simulink model "TV_2021"  (R2017b)
settings: Solver=VariableStepAuto  StartTime=0.0  StopTime=10.0  RelTol=1e-3
undefined symbols (not defined in the file): sigbuilder_block
libraries: simulink x6
(part 7 of 13)

== system TV_2021/Vehicle Dynamics Control 1/VDC 2018 without Longitudinal/Driver // CarBehaviours/Accelerating ==
  Throttle : Inport
  Tq_RR : Inport  Port=2
  "Tq_RL " : Inport  Port=3
  Action Port : ActionPort
  Product : Product
  Product1 : Product
  "Tq_RR " : Outport
  Tq_RL : Outport  Port=2
  Out_Throttle : Outport  Port=3
  wires:
  "Tq_RL "/1 -> Product/2
  Tq_RR/1 -> Product1/2
  Throttle/1 -> Product1/1, Product/1, Out_Throttle/1
  Product/1 -> Tq_RL/1
  Product1/1 -> "Tq_RR "/1

== system TV_2021/Vehicle Dynamics Control 1/VDC 2018 without Longitudinal/Driver // CarBehaviours/Inertia Braking ==
  Action Port : ActionPort
  Constant : Constant  Value=0
  Constant1 : Constant  Value=0
  "Tq_RR " : Outport
  Tq_RL : Outport  Port=2
  wires:
  Constant/1 -> "Tq_RR "/1
  Constant1/1 -> Tq_RL/1

== system TV_2021/Vehicle Dynamics Control 1/VDC 2018 without Longitudinal/Driver // CarBehaviours/Mech_Braking ==
  Action Port : ActionPort
  Constant : Constant  Value=0
  Constant1 : Constant  Value=0
  "Tq_RR " : Outport
  Tq_RL : Outport  Port=2
  wires:
  Constant/1 -> "Tq_RR "/1
  Constant1/1 -> Tq_RL/1

== system TV_2021/Vehicle Dynamics Control 1/VDC 2018 without Longitudinal/Driver // CarBehaviours/Regenerative+Mech Braking ==
  RegTq_RR : Inport
  RegTq_RL : Inport  Port=2
  Action Port : ActionPort
  "Tq_RR " : Outport
  Tq_RL : Outport  Port=2
  wires:
  RegTq_RL/1 -> Tq_RL/1
  RegTq_RR/1 -> "Tq_RR "/1

== system TV_2021/Vehicle Dynamics Control 1/VDC 2018 without Longitudinal/Optimization SKF & CKF/Subsystem  ==
  Derivative : Inport
  "CKF_Initial " : Inport  Port=2
  "CKF_prev " : Inport  Port=3
  Cte_CKF : Inport  Port=4
  CKF : Subsystem
  CKF_act : Outport
  wires:
  Cte_CKF/1 -> CKF/4(Cte_CKF)
  "CKF_Initial "/1 -> CKF/2(CKF_Initial)
  Derivative/1 -> CKF/1(Derivative)
  "CKF_prev "/1 -> CKF/3("CKF_prev ")
  CKF/1("CKF_act ") -> CKF_act/1

== system TV_2021/Vehicle Dynamics Control 1/VDC 2018 without Longitudinal/Wheel_to_engine/Fx_to_engineTqRL ==
  Fx : Inport
  Re : Inport  Port=2
  RT : Inport  Port=3
  Divide : Product  Inputs=*/
  Product : Product
  Tq : Outport
  wires:
  Re/1 -> Product/2
  Fx/1 -> Product/1
  RT/1 -> Divide/2
  Product/1 -> Divide/1
  Divide/1 -> Tq/1

== system TV_2021/Vehicle Dynamics Control 1/VDC 2018 without Longitudinal/Wheel_to_engine/Fx_to_engineTqRR ==
  Fx : Inport
  Re : Inport  Port=2
  RT : Inport  Port=3
  Divide : Product  Inputs=*/
  Product : Product
  Tq : Outport
  wires:
  Re/1 -> Product/2
  Fx/1 -> Product/1
  RT/1 -> Divide/2
  Product/1 -> Divide/1
  Divide/1 -> Tq/1

== system TV_2021/Vehicle Dynamics Control 2018/Steering TV 2017 with TC/Constraints/Control de Potencia  ==
  Tq_RR : Inport
  Tq_RL : Inport  Port=2
  ReductionCte : Inport  Port=3
  Action Port : ActionPort
  Add : Sum  Inputs=+-
  Add1 : Sum  Inputs=+-
  Product : Product
  Product1 : Product
  Tq_RR_out : Outport
  Tq_RL_out : Outport  Port=2
  wires:
  Tq_RR/1 -> Product/1, Add/1
  Tq_RL/1 -> Product1/1, Add1/1
  ReductionCte/1 -> Product/2, Product1/2
  Product1/1 -> Add1/2
  Product/1 -> Add/2
  Add1/1 -> Tq_RL_out/1
  Add/1 -> Tq_RR_out/1

== system TV_2021/Vehicle Dynamics Control 2018/Steering TV 2017 with TC/Constraints/Control de Temperatura ==
  Tq_RR : Inport
  Tq_RL : Inport  Port=2
  ReductionCte : Inport  Port=3
  Action Port : ActionPort
  Add : Sum  Inputs=+-
  Add1 : Sum  Inputs=+-
  Product : Product
  Product1 : Product
  Tq_RR_out : Outport
  Tq_RL_out : Outport  Port=2
  wires:
  Product/1 -> Add/2
  Product1/1 -> Add1/2
  Add1/1 -> Tq_RL_out/1
  Tq_RR/1 -> Add/1, Product/1
  Tq_RL/1 -> Add1/1, Product1/1
  ReductionCte/1 -> Product1/2, Product/2
  Add/1 -> Tq_RR_out/1

== system TV_2021/Vehicle Dynamics Control 2018/Steering TV 2017 with TC/Constraints/current_limitation1 ==
  note: % de la corriente total que te dejo usar
  max_cell_temp : Inport
  actual_current : Inport  Port=2
  initial_limitation : Inport  Port=3
  max_discharge_current : Inport  Port=4
  max_regen_current : Inport  Port=5
  Product1 : Product
  constants_saturator : Subsystem
  temperature_rise_limitator : Subsystem
  max_discharge (-) : Outport  VectorParamsAs1DForOutWhenUnconnected=on
  max_regen (+) : Outport  Port=2  VectorParamsAs1DForOutWhenUnconnected=on
  fans_control : Outport  Port=3  VectorParamsAs1DForOutWhenUnconnected=on
  wires:
  actual_current/1 -> Product1/2
  max_cell_temp/1 -> temperature_rise_limitator/1(max_cell_temp)
  Product1/1 -> constants_saturator/1(allowed_current [%])
  constants_saturator/1(limited_discharge_actual) -> max_discharge (-)/1
  constants_saturator/2(limited_regen_actual) -> max_regen (+)/1
  initial_limitation/1 -> temperature_rise_limitator/2(initial_limitation)
  max_discharge_current/1 -> constants_saturator/2(max_discharge_current)
  max_regen_current/1 -> constants_saturator/3(max_regen_current)
  temperature_rise_limitator/1(allowed_current) -> fans_control/1, Product1/1

== system TV_2021/Vehicle Dynamics Control 2018/Steering TV 2017 with TC/Constraints/else ==
  Tq_RR : Inport
  Tq_RL : Inport  Port=2
  Action Port : ActionPort
  Tq_RR_out : Outport
  Tq_RL_out : Outport  Port=2
  wires:
  Tq_RR/1 -> Tq_RR_out/1
  Tq_RL/1 -> Tq_RL_out/1

== system TV_2021/Vehicle Dynamics Control 2018/Steering TV 2017 with TC/Optimization SKF & CKF/Subsystem  ==
  Steer_An : Inport
  Derivative : Inport  Port=2
  SKF_Initial : Inport  Port=3
  SKF_prev : Inport  Port=4
  "CKF_Initial " : Inport  Port=5
  "CKF_prev " : Inport  Port=6
  Cte_SKF : Inport  Port=7
  Cte_CKF : Inport  Port=8
  CKF : Subsystem
  MATLAB Function1 : MATLAB Function  TreatAsAtomicUnit=on
  SKF : Subsystem
  SKF or CKF : If  IfExpression=-10 < u1 & u1 < 10
  Steering Wheel Maximum Angle : Constant  Value=100
  "SKF_act " : Outport
  CKF_act : Outport  Port=2
  wires:
  MATLAB Function1/1(value) -> SKF or CKF/1
  Steering Wheel Maximum Angle/1 -> MATLAB Function1/1(cte)
  Steer_An/1 -> MATLAB Function1/2(v)
  SKF/1(SKF_act) -> "SKF_act "/1
  CKF/1("CKF_act ") -> CKF_act/1
  SKF or CKF/1 -> SKF/Action
  SKF or CKF/2 -> CKF/Action
  "CKF_prev "/1 -> CKF/3("CKF_prev ")
  Derivative/1 -> CKF/1(Derivative), SKF/1(Derivative)
  SKF_Initial/1 -> SKF/2("SKF_Initial ")
  SKF_prev/1 -> SKF/3(SKF_prev)
  "CKF_Initial "/1 -> CKF/2(CKF_Initial)
  Cte_SKF/1 -> SKF/4(Cte_SKF)
  Cte_CKF/1 -> CKF/4(Cte_CKF)

== system TV_2021/Vehicle Dynamics Control 2018/VDC 2018 Complete/Constraints/Acelerating and braking without Regenerative ==
  Tq_max : Inport
  V_eRR : Inport  Port=2
  V_eRL : Inport  Port=3
  Trans_max_dynamic : Inport  Port=4
  Trans_max_static : Inport  Port=5
  Power_limit : Inport  Port=6
  Power : Inport  Port=7
  Temperature_limit_IGBT : Inport  Port=8
  TemperatureIGBT : Inport  Port=9
  TemperatureI_limit_Motor : Inport  Port=10
  TemperatureMotor : Inport  Port=11
  ReductionCte_Power : Inport  Port=12
  ReductionCte_Temperature : Inport  Port=13
  Tq_FR : Inport  Port=14
  Tq_FL : Inport  Port=15
  Tq_RR : Inport  Port=16
  Tq_RL : Inport  Port=17
  Tq_diff : Inport  Port=18
  Tq_diff_max : Inport  Port=19
  Temp_celdas : Inport  Port=20
  Limit_Temp_celdas : Inport  Port=21
  Action Port : ActionPort
  "Control de Potencia " : Subsystem  TreatAsAtomicUnit=on
  Control de Temperatura : Subsystem  TreatAsAtomicUnit=on
  Gain : Gain  Gain=3.141592/30
  If : If  NumInputs=8  IfExpression=u4 >= u3 | u6 >= u5 | u7>=u8  ElseIfExpressions=u2 >= u1
  If Action 1 : Subsystem  TreatAsAtomicUnit=on
  If Action 2 : Subsystem  TreatAsAtomicUnit=on
  If1 : If  NumInputs=3  IfExpression=u1 > u3 & u2 > u3
  MATLAB Function : MATLAB Function  TreatAsAtomicUnit=on
  Merge{,1,3..4} (4 alike) : Merge  Inputs=3
  Merge2 : Merge
  Momentum Z scaled : Subsystem
  Terminator : Terminator
  Terminator1 : Terminator
  else : Subsystem  TreatAsAtomicUnit=on
  minimum value : MATLAB Function  TreatAsAtomicUnit=on
  minimum value1 : MATLAB Function  TreatAsAtomicUnit=on
  rpm : Constant  Value=200
  TQ_RR : Outport
  TQ_RL : Outport  Port=2
  Flag_Temperature : Outport  Port=3
  Flag_Power : Outport  Port=4
  wires:
  If1/1 -> If Action 1/Action
  If Action 1/1(Trans_limit) -> Merge2/1
  Merge2/1 -> minimum value/1(a), minimum value1/1(a)
  Trans_max_dynamic/1 -> If Action 1/1(Trans_max_dynamic)
  If Action 2/1(Trans_limit) -> Merge2/2
  V_eRR/1 -> If1/1
  V_eRL/1 -> If1/2
  If1/2 -> If Action 2/Action
  Trans_max_static/1 -> If Action 2/1("Trans_max_static ")
  Tq_max/1 -> minimum value1/2(b), minimum value/2(b)
  rpm/1 -> Gain/1
  Gain/1 -> If1/3  "approx 20.95"
  Tq_FR/1 -> Terminator/1
  Tq_FL/1 -> Terminator1/1
  TemperatureIGBT/1 -> If/4
  ReductionCte_Power/1 -> "Control de Potencia "/3(ReductionCte)
  If/3 -> else/Action
  Power_limit/1 -> If/1
  Power/1 -> If/2
  Temperature_limit_IGBT/1 -> If/3
  minimum value/1(min) -> Control de Temperatura/1(Tq_RR), "Control de Potencia "/1(Tq_RR), else/1(Tq_RR)
  minimum value1/1(min) -> Control de Temperatura/2(Tq_RL), "Control de Potencia "/2(Tq_RL), else/2(Tq_RL)
  ReductionCte_Temperature/1 -> Control de Temperatura/3(ReductionCte)
  "Control de Potencia "/1(Tq_RR_out) -> Merge/1
  Control de Temperatura/1(Tq_RR_out) -> Merge/2
  else/1(Tq_RR_out) -> Merge/3
  "Control de Potencia "/2(Tq_RL_out) -> Merge1/1
  Control de Temperatura/2(Tq_RL_out) -> Merge1/2
  else/2(Tq_RL_out) -> Merge1/3
  If/1 -> Control de Temperatura/Action
  If/2 -> "Control de Potencia "/Action
  Tq_RR/1 -> [tq_RR_wc], minimum value/3(c)
  Tq_RL/1 -> [tq_RL_wc], minimum value1/3(c)
  Merge/1 -> Momentum Z scaled/1(Tq_RR_Lim)
  Merge1/1 -> Momentum Z scaled/2(Tq_RL_Lim)
  [tq_RR_wc] -> Momentum Z scaled/3(Tq_RR_wc)
  [tq_RL_wc] -> Momentum Z scaled/4(Tq_RL_wc)
  TemperatureI_limit_Motor/1 -> If/5
  TemperatureMotor/1 -> If/6
  Merge3/1 -> Flag_Temperature/1
  Merge4/1 -> Flag_Power/1
  Control de Temperatura/3(Flag_Temperature) -> Merge3/1
  Control de Temperatura/4(Flag_Power) -> Merge4/1
  "Control de Potencia "/3(Flag_Temperature) -> Merge3/2
  "Control de Potencia "/4(Flag_Power) -> Merge4/2
  else/3(Flag_Temperature) -> Merge3/3
  else/4(Flag_Power) -> Merge4/3
  Momentum Z scaled/1(TQ_RR) -> TQ_RR/1
  Momentum Z scaled/2(TQ_RL) -> TQ_RL/1
  Tq_diff/1 -> MATLAB Function/1(diff_wc)
  Tq_diff_max/1 -> MATLAB Function/2(diff_max)
  MATLAB Function/1(diff_lim) -> [Tq_diff_lim]
  [Tq_diff_lim] -> Momentum Z scaled/5(Tq_diff)
  Temp_celdas/1 -> If/7
  Limit_Temp_celdas/1 -> If/8

== system TV_2021/Vehicle Dynamics Control 2018/VDC 2018 Complete/Constraints/Braking with Regenerative ==
  MaxRegTorque : Inport
  Tq_RR_wc : Inport  Port=2
  Tq_RL_wc : Inport  Port=3
  Action Port : ActionPort
  Gain : Gain  Gain=-1
  Gain1 : Gain  Gain=-1
  MATLAB Function : MATLAB Function  TreatAsAtomicUnit=on
  TQ_RR : Outport
  TQ_RL : Outport  Port=2
  wires:
  MATLAB Function/2(RegTq_RL) -> Gain1/1
  MATLAB Function/1(RegTq_RR) -> Gain/1
  Tq_RR_wc/1 -> MATLAB Function/2(Tq_RR)
  Tq_RL_wc/1 -> MATLAB Function/3(Tq_RL)
  MaxRegTorque/1 -> MATLAB Function/1(MaxRegenTq)
  Gain1/1 -> TQ_RL/1
  Gain/1 -> TQ_RR/1

== system TV_2021/Vehicle Dynamics Control 2018/VDC 2018 Complete/Driver // CarBehaviours/Accelerating ==
  Throttle : Inport
  Tq_RR : Inport  Port=2
  "Tq_RL " : Inport  Port=3
  Action Port : ActionPort
  Product : Product
  Product1 : Product
  "Tq_RR " : Outport
  Tq_RL : Outport  Port=2
  Out_Throttle : Outport  Port=3
  wires:
  Product1/1 -> "Tq_RR "/1
  Product/1 -> Tq_RL/1
  Throttle/1 -> Out_Throttle/1, Product/1, Product1/1
  Tq_RR/1 -> Product1/2
  "Tq_RL "/1 -> Product/2

== system TV_2021/Vehicle Dynamics Control 2018/VDC 2018 Complete/Driver // CarBehaviours/Inertia Braking ==
  Action Port : ActionPort
  Constant : Constant  Value=0
  Constant1 : Constant  Value=0
  "Tq_RR " : Outport
  Tq_RL : Outport  Port=2
  wires:
  Constant1/1 -> Tq_RL/1
  Constant/1 -> "Tq_RR "/1

== system TV_2021/Vehicle Dynamics Control 2018/VDC 2018 Complete/Driver // CarBehaviours/Mech_Braking ==
  Action Port : ActionPort
  Constant : Constant  Value=0
  Constant1 : Constant  Value=0
  "Tq_RR " : Outport
  Tq_RL : Outport  Port=2
  wires:
  Constant1/1 -> Tq_RL/1
  Constant/1 -> "Tq_RR "/1

== system TV_2021/Vehicle Dynamics Control 2018/VDC 2018 Complete/Driver // CarBehaviours/Regenerative+Mech Braking ==
  RegTq_RR : Inport
  RegTq_RL : Inport  Port=2
  Action Port : ActionPort
  "Tq_RR " : Outport
  Tq_RL : Outport  Port=2
  wires:
  RegTq_RR/1 -> "Tq_RR "/1
  RegTq_RL/1 -> Tq_RL/1

== system TV_2021/Vehicle Dynamics Control 2018/VDC 2018 Complete/Lateral Dynamics/Kamm_Circle ==
  Fz_R : Inport
  Fz_L : Inport  Port=2
  Fy : Inport  Port=3
  CK_Factor : Inport  Port=4
  Kamm_Circle LatD : MATLAB Function  TreatAsAtomicUnit=on
  Product1 : Product
  Product2 : Product
  Fx_R : Outport
  Fx_L : Outport  Port=2
  Fy_R [N] (0,inf) : Outport  Port=3
  wires:
  Kamm_Circle LatD/3(Fy_R) -> Fy_R [N] (0,inf)/1
  Fz_L/1 -> Kamm_Circle LatD/2(Fz_L)
  Fz_R/1 -> Kamm_Circle LatD/1(Fz_R)
  Fy/1 -> Kamm_Circle LatD/3(Fy)
  Kamm_Circle LatD/1(Fx_R) -> Product1/1
  Kamm_Circle LatD/2(Fx_L) -> Product2/1
  Product2/1 -> Fx_L/1
  CK_Factor/1 -> Product2/2, Product1/2
  Product1/1 -> Fx_R/1

== system TV_2021/Vehicle Dynamics Control 2018/VDC 2018 Complete/Lateral Dynamics/Tire Longitudinal Force Difference ==
  e : Inport
  Iz : Inport  Port=2
  dt : Inport  Port=3
  rt : Inport  Port=4
  " Momentum_Z to Longitudinal Force Difference" : Subsystem
  Momentum respect to Z-axis to correct the error : Subsystem
  Scope5 : Scope
  Scope6 : Scope
  Fx_diff : Outport
  wires:
  dt/1 -> Momentum respect to Z-axis to correct the error/3(Correction_Time [s])
  rt/1 -> " Momentum_Z to Longitudinal Force Difference"/2(RearTrackwidth [m])
  " Momentum_Z to Longitudinal Force Difference"/1(Fx_diff [N]) -> Fx_diff/1
  Iz/1 -> Momentum respect to Z-axis to correct the error/2(Iz [kg/m^3])
  Momentum respect to Z-axis to correct the error/1(Momentum_Z [Nm]) -> " Momentum_Z to Longitudinal Force Difference"/1("\tMomentumZ [Nm]"), Scope6/1
  e/1 -> Scope5/1, Momentum respect to Z-axis to correct the error/1(Yaw_error_[º/s])

== system TV_2021/Vehicle Dynamics Control 2018/VDC 2018 Complete/Lateral Dynamics/Yaw_Rate_Reference ==
  Steering_Angle : Inport
  F_vel_x : Inport  Port=2
  360/(2*pi) : Gain  Gain=360/(2*pi)
  360/(2pi) : Gain  Gain=360/(2*pi)
  Bicycle Model : MATLAB Function  TreatAsAtomicUnit=on
  Constant7 : Constant  Value=0.92
  Constant8 : Constant  Value=360
  Cornering_Stiffness_F[N/º] : Constant  Value=-700
  Cornering_Stiffness_R[N/º] : Constant  Value=-1000
  Divide : Product  Inputs=*/
  Gain{,1..4} (5 alike) : Gain  Gain=360/(2*pi)
  Scope1 : Scope  NumInputPorts=5
  Scope2 : Scope  NumInputPorts=2
  Scope3 : Scope
  Steering_Ratio [-] : Constant  Value=3.72
  Wheelbase [m] : Constant  Value=1.53
  Yaw_Rate : Outport
  wires:
  Gain4/1 -> Scope1/2
  Gain3/1 -> Scope1/3
  Gain2/1 -> Scope1/4
  Gain1/1 -> Scope1/1
  Gain/1 -> Scope1/5
  360/(2pi)/1 -> Bicycle Model/7(cr)
  Cornering_Stiffness_R[N/º]/1 -> 360/(2pi)/1
  360/(2*pi)/1 -> Bicycle Model/6(cf)
  Bicycle Model/2(beta) -> Gain2/1
  F_vel_x/1 -> Bicycle Model/2(vx)
  Bicycle Model/7(yf) -> Scope2/1
  Bicycle Model/3(alpha_f) -> Gain4/1
  Bicycle Model/6(radius) -> Scope3/1
  Cornering_Stiffness_F[N/º]/1 -> 360/(2*pi)/1
  Constant7/1 -> Bicycle Model/4(xCG)
  Bicycle Model/5(course) -> Gain/1
  Constant8/1 -> Bicycle Model/3(m)
  Bicycle Model/4(alpha_r) -> Gain3/1
  Steering_Ratio [-]/1 -> Divide/2
  Bicycle Model/1(r) -> Yaw_Rate/1
  Divide/1 -> Gain1/1, Bicycle Model/1(delta)
  Wheelbase [m]/1 -> Bicycle Model/5(L)
  Steering_Angle/1 -> Divide/1
  Bicycle Model/8(yr) -> Scope2/2

== system TV_2021/Vehicle Dynamics Control 2018/VDC 2018 Complete/Longitudinal Dynamics/Kamm_Circle ==
  Fz_R : Inport
  Fz_L : Inport  Port=2
  Fy : Inport  Port=3
  SK_Factor : Inport  Port=4
  Kamm_Circle LatD : MATLAB Function  TreatAsAtomicUnit=on
  Product : Product
  Product1 : Product
  Fx_R : Outport
  Fx_L : Outport  Port=2
  wires:
  Kamm_Circle LatD/1(Fx_R) -> Product/1
  Kamm_Circle LatD/2(Fx_L) -> Product1/1
  Fz_L/1 -> Kamm_Circle LatD/2(Fz_L)
  Fy/1 -> Kamm_Circle LatD/3(Fy)
  SK_Factor/1 -> Product/2, Product1/2
  Product/1 -> Fx_R/1
  Product1/1 -> Fx_L/1
  Fz_R/1 -> Kamm_Circle LatD/1(Fz_R)

== system TV_2021/Vehicle Dynamics Control 2018/VDC 2018 Complete/Optimization SKF & CKF/Subsystem  ==
  Steer_An : Inport
  Derivative : Inport  Port=2
  SKF_Initial : Inport  Port=3
  SKF_prev : Inport  Port=4
  "CKF_Initial " : Inport  Port=5
  "CKF_prev " : Inport  Port=6
  Cte_SKF : Inport  Port=7
  Cte_CKF : Inport  Port=8
  CKF : Subsystem
  MATLAB Function1 : MATLAB Function  TreatAsAtomicUnit=on
  SKF : Subsystem
  SKF or CKF : If  IfExpression=-10 < u1 & u1 < 10
  Steering Wheel Maximum Angle : Constant  Value=100
  "SKF_act " : Outport
  CKF_act : Outport  Port=2
  wires:
  MATLAB Function1/1(value) -> SKF or CKF/1
  Steering Wheel Maximum Angle/1 -> MATLAB Function1/1(cte)
  Steer_An/1 -> MATLAB Function1/2(v)
  SKF/1(SKF_act) -> "SKF_act "/1
  CKF/1("CKF_act ") -> CKF_act/1
  SKF or CKF/1 -> SKF/Action
  SKF or CKF/2 -> CKF/Action
  "CKF_prev "/1 -> CKF/3("CKF_prev ")
  Derivative/1 -> CKF/1(Derivative), SKF/1(Derivative)
  SKF_Initial/1 -> SKF/2("SKF_Initial ")
  SKF_prev/1 -> SKF/3(SKF_prev)
  "CKF_Initial "/1 -> CKF/2(CKF_Initial)
  Cte_SKF/1 -> SKF/4(Cte_SKF)
  Cte_CKF/1 -> CKF/4(Cte_CKF)

== system TV_2021/Vehicle Dynamics Control 2018/VDC 2018 Complete/Wheel_to_engine/Fx_to_engineTqRL ==
  Fx : Inport
  Re : Inport  Port=2
  RT : Inport  Port=3
  Divide : Product  Inputs=*/
  Product : Product
  Tq : Outport
  wires:
  Divide/1 -> Tq/1
  Product/1 -> Divide/1
  RT/1 -> Divide/2
  Fx/1 -> Product/1
  Re/1 -> Product/2

== system TV_2021/Vehicle Dynamics Control 2018/VDC 2018 Complete/Wheel_to_engine/Fx_to_engineTqRR ==
  Fx : Inport
  Re : Inport  Port=2
  RT : Inport  Port=3
  Divide : Product  Inputs=*/
  Product : Product
  Tq : Outport
  wires:
  Divide/1 -> Tq/1
  Product/1 -> Divide/1
  RT/1 -> Divide/2
  Fx/1 -> Product/1
  Re/1 -> Product/2

== system TV_2021/Vehicle Dynamics Control 2018/VDC 2018 without Longitudinal/Constraints/Acelerating and braking without Regenerative ==
  note: Considero de la misma gravedad,
      | la limitacion por potencia que por temperatura
  Tq_max : Inport
  V_eRR : Inport  Port=2
  V_eRL : Inport  Port=3
  Trans_max_dynamic : Inport  Port=4
  Trans_max_static : Inport  Port=5
  Tq_FR : Inport  Port=6
  Tq_FL : Inport  Port=7
  Tq_RR : Inport  Port=8
  Tq_RL : Inport  Port=9
  Power_limit1 : Inport  Port=10
  Power1 : Inport  Port=11
  Temperature_limit_IGBT1 : Inport  Port=12
  Temperature_IGBT : Inport  Port=13
  Temperature_limit_Motor : Inport  Port=14
  Temperature_Motor : Inport  Port=15
  Temp_Celdas : Inport  Port=16
  Lim_Temp_Celdas : Inport  Port=17
  ReductionCte_Temperature1 : Inport  Port=18
  ReductionCte_Power1 : Inport  Port=19
  Action Port : ActionPort
  Control de Potencia 1 : Subsystem  TreatAsAtomicUnit=on
  Control de Temperatura1 : Subsystem  TreatAsAtomicUnit=on
  Gain : Gain  Gain=3.141592/30
  If Action 1 : Subsystem  TreatAsAtomicUnit=on
  If Action 2 : Subsystem  TreatAsAtomicUnit=on
  If1 : If  NumInputs=3  IfExpression=u1 > u3 & u2 > u3
  If2 : If  NumInputs=8  IfExpression=u4 >= u3 | u6 >= u5 | u7>=u8  ElseIfExpressions=u2 >= u1
  Merge2 : Merge
  Merge3 : Merge  Inputs=3
  Merge4 : Merge  Inputs=3
  Momentum Z scaled : Subsystem
  Terminator : Terminator
  Terminator1 : Terminator
  else1 : Subsystem  TreatAsAtomicUnit=on
  minimum value : MATLAB Function  TreatAsAtomicUnit=on
  minimum value1 : MATLAB Function  TreatAsAtomicUnit=on
  rpm : Constant  Value=200
  TQ_RR : Outport
  TQ_RL : Outport  Port=2
  wires:
  If1/1 -> If Action 1/Action
  If Action 1/1(Trans_limit) -> Merge2/1
  Merge2/1 -> minimum value/1(a), minimum value1/1(a)
  Trans_max_dynamic/1 -> If Action 1/1(Trans_max_dynamic)
  If Action 2/1(Trans_limit) -> Merge2/2
  V_eRR/1 -> If1/1
  V_eRL/1 -> If1/2
  If1/2 -> If Action 2/Action
  Trans_max_static/1 -> If Action 2/1("Trans_max_static ")
  Tq_max/1 -> minimum value1/2(b), minimum value/2(b)
  rpm/1 -> Gain/1
  Gain/1 -> If1/3  "approx 20.95"
  Tq_FR/1 -> Terminator/1
  Tq_FL/1 -> Terminator1/1
  Tq_RR/1 -> [tq_RR_wc], minimum value/3(c)
  Tq_RL/1 -> [tq_RL_wc], minimum value1/3(c)
  Merge3/1 -> Momentum Z scaled/1(Tq_RR_Lim)
  Merge4/1 -> Momentum Z scaled/2(Tq_RL_Lim)
  [tq_RR_wc] -> Momentum Z scaled/3(Tq_RR_wc)
  [tq_RL_wc] -> Momentum Z scaled/4(Tq_RL_wc)
  Momentum Z scaled/1(TQ_RR) -> TQ_RR/1
  Momentum Z scaled/2(TQ_RL) -> TQ_RL/1
  Temp_Celdas/1 -> If2/7
  Lim_Temp_Celdas/1 -> If2/8
  Control de Temperatura1/1(Tq_RR_out) -> Merge3/2
  Temperature_limit_Motor/1 -> If2/5
  Temperature_Motor/1 -> If2/6
  else1/1(Tq_RR_out) -> Merge3/3
  Control de Temperatura1/2(Tq_RL_out) -> Merge4/2
  If2/2 -> Control de Potencia 1/Action
  If2/3 -> else1/Action
  else1/2(Tq_RL_out) -> Merge4/3
  minimum value/1(min) -> Control de Temperatura1/1(Tq_RR), Control de Potencia 1/1(Tq_RR), else1/1(Tq_RR)
  Control de Potencia 1/1(Tq_RR_out) -> Merge3/1
  ReductionCte_Temperature1/1 -> Control de Temperatura1/3(ReductionCte)
  If2/1 -> Control de Temperatura1/Action
  Temperature_limit_IGBT1/1 -> If2/3
  Power1/1 -> If2/2
  ReductionCte_Power1/1 -> Control de Potencia 1/3(ReductionCte)
  minimum value1/1(min) -> Control de Temperatura1/2(Tq_RL), Control de Potencia 1/2(Tq_RL), else1/2(Tq_RL)
  Temperature_IGBT/1 -> If2/4
  Control de Potencia 1/2(Tq_RL_out) -> Merge4/1
  Power_limit1/1 -> If2/1

== system TV_2021/Vehicle Dynamics Control 2018/VDC 2018 without Longitudinal/Constraints/Braking with Regenerative ==
  MaxRegTorque : Inport
  Tq_RR_wc : Inport  Port=2
  Tq_RL_wc : Inport  Port=3
  Action Port : ActionPort
  Gain : Gain  Gain=-1
  Gain1 : Gain  Gain=-1
  MATLAB Function : MATLAB Function  TreatAsAtomicUnit=on
  TQ_RR : Outport
  TQ_RL : Outport  Port=2
  wires:
  MATLAB Function/2(RegTq_RL) -> Gain1/1
  MATLAB Function/1(RegTq_RR) -> Gain/1
  Tq_RR_wc/1 -> MATLAB Function/2(Tq_RR)
  Tq_RL_wc/1 -> MATLAB Function/3(Tq_RL)
  MaxRegTorque/1 -> MATLAB Function/1(MaxRegenTq)
  Gain1/1 -> TQ_RL/1
  Gain/1 -> TQ_RR/1

== system TV_2021/Vehicle Dynamics Control 2018/VDC 2018 without Longitudinal/Driver // CarBehaviours/Accelerating ==
  Throttle : Inport
  Tq_RR : Inport  Port=2
  "Tq_RL " : Inport  Port=3
  Action Port : ActionPort
  Product : Product
  Product1 : Product
  "Tq_RR " : Outport
  Tq_RL : Outport  Port=2
  Out_Throttle : Outport  Port=3
  wires:
  Product1/1 -> "Tq_RR "/1
  Product/1 -> Tq_RL/1
  Throttle/1 -> Out_Throttle/1, Product/1, Product1/1
  Tq_RR/1 -> Product1/2
  "Tq_RL "/1 -> Product/2

== system TV_2021/Vehicle Dynamics Control 2018/VDC 2018 without Longitudinal/Driver // CarBehaviours/Inertia Braking ==
  Action Port : ActionPort
  Constant : Constant  Value=0
  Constant1 : Constant  Value=0
  "Tq_RR " : Outport
  Tq_RL : Outport  Port=2
  wires:
  Constant1/1 -> Tq_RL/1
  Constant/1 -> "Tq_RR "/1

== system TV_2021/Vehicle Dynamics Control 2018/VDC 2018 without Longitudinal/Driver // CarBehaviours/Mech_Braking ==
  Action Port : ActionPort
  Constant : Constant  Value=0
  Constant1 : Constant  Value=0
  "Tq_RR " : Outport
  Tq_RL : Outport  Port=2
  wires:
  Constant1/1 -> Tq_RL/1
  Constant/1 -> "Tq_RR "/1

== system TV_2021/Vehicle Dynamics Control 2018/VDC 2018 without Longitudinal/Driver // CarBehaviours/Regenerative+Mech Braking ==
  RegTq_RR : Inport
  RegTq_RL : Inport  Port=2
  Action Port : ActionPort
  "Tq_RR " : Outport
  Tq_RL : Outport  Port=2
  wires:
  RegTq_RR/1 -> "Tq_RR "/1
  RegTq_RL/1 -> Tq_RL/1

== system TV_2021/Vehicle Dynamics Control 2018/VDC 2018 without Longitudinal/Optimization SKF & CKF/Subsystem  ==
  Derivative : Inport
  "CKF_Initial " : Inport  Port=2
  "CKF_prev " : Inport  Port=3
  Cte_CKF : Inport  Port=4
  CKF : Subsystem
  CKF_act : Outport
  wires:
  CKF/1("CKF_act ") -> CKF_act/1
  "CKF_prev "/1 -> CKF/3("CKF_prev ")
  Derivative/1 -> CKF/1(Derivative)
  "CKF_Initial "/1 -> CKF/2(CKF_Initial)
  Cte_CKF/1 -> CKF/4(Cte_CKF)

== system TV_2021/Vehicle Dynamics Control 2018/VDC 2018 without Longitudinal/Wheel_to_engine/Fx_to_engineTqRL ==
  Fx : Inport
  Re : Inport  Port=2
  RT : Inport  Port=3
  Divide : Product  Inputs=*/
  Product : Product
  Tq : Outport
  wires:
  Divide/1 -> Tq/1
  Product/1 -> Divide/1
  RT/1 -> Divide/2
  Fx/1 -> Product/1
  Re/1 -> Product/2

== system TV_2021/Vehicle Dynamics Control 2018/VDC 2018 without Longitudinal/Wheel_to_engine/Fx_to_engineTqRR ==
  Fx : Inport
  Re : Inport  Port=2
  RT : Inport  Port=3
  Divide : Product  Inputs=*/
  Product : Product
  Tq : Outport
  wires:
  Divide/1 -> Tq/1
  Product/1 -> Divide/1
  RT/1 -> Divide/2
  Fx/1 -> Product/1
  Re/1 -> Product/2

== system TV_2021/If Action Subsystem1/Steering TV 2017 with TC/Optimization SKF & CKF/Subsystem /CKF ==
  Derivative : Inport
  CKF_Initial : Inport  Port=2
  "CKF_prev " : Inport  Port=3
  Cte_CKF : Inport  Port=4
  Action Port : ActionPort
  If1 : If  IfExpression=u1 >= 900  ElseIfExpressions=u1 < 900  ShowElse=off
  Merge : Merge
  No spin : Subsystem  TreatAsAtomicUnit=on
  Saturation : Saturate  UpperLimit=1  LowerLimit=0.3
  "Spin " : Subsystem  TreatAsAtomicUnit=on
  "CKF_act " : Outport
  wires:
  Merge/1 -> Saturation/1
  "CKF_prev "/1 -> "Spin "/1(CKF_prev), No spin/2(CKF_prev)
  If1/1 -> "Spin "/Action
  Derivative/1 -> If1/1
  Cte_CKF/1 -> "Spin "/3(Cte_CKF)
  "Spin "/1("CKF_act1 ") -> Merge/2
  Saturation/1 -> "CKF_act "/1
  CKF_Initial/1 -> "Spin "/2("CKF_Initial "), No spin/1(CKF_Initial)
  If1/2 -> No spin/Action
  No spin/1(CKF_act0) -> Merge/1

== system TV_2021/If Action Subsystem1/Steering TV 2017 with TC/Optimization SKF & CKF/Subsystem /SKF ==
  Derivative : Inport
  "SKF_Initial " : Inport  Port=2
  SKF_prev : Inport  Port=3
  Cte_SKF : Inport  Port=4
  Action Port : ActionPort
  If : If  IfExpression=u1 >=900  ElseIfExpressions=u1 < 900  ShowElse=off
  Merge : Merge
  No spin : Subsystem  TreatAsAtomicUnit=on
  Saturation : Saturate  UpperLimit=1  LowerLimit=0.3
  Spin : Subsystem  TreatAsAtomicUnit=on
  SKF_act : Outport
  wires:
  Merge/1 -> Saturation/1
  Derivative/1 -> If/1
  Spin/1(SKF_act1) -> Merge/2
  "SKF_Initial "/1 -> Spin/1(SKF_Initial), No spin/1(SKF_Initial)
  No spin/1(SKF_act0) -> Merge/1
  If/2 -> No spin/Action
  SKF_prev/1 -> Spin/2(SKF_prev), No spin/2(SKF_prev)
  Cte_SKF/1 -> Spin/3(Cte_SKF)
  Saturation/1 -> SKF_act/1
  If/1 -> Spin/Action

== system TV_2021/If Action Subsystem1/VDC 2018 Complete/Constraints/Acelerating and braking without Regenerative/Control de Potencia  ==
  Tq_RR : Inport
  Tq_RL : Inport  Port=2
  ReductionCte : Inport  Port=3
  Action Port : ActionPort
  Add : Sum  Inputs=+-
  Add1 : Sum  Inputs=+-
  Constant : Constant  Value=0
  Constant1 : Constant
  Product : Product
  Product1 : Product
  Tq_RR_out : Outport
  Tq_RL_out : Outport  Port=2
  Flag_Temperature : Outport  Port=3
  Flag_Power : Outport  Port=4
  wires:
  Tq_RR/1 -> Product/1, Add/1
  Tq_RL/1 -> Product1/1, Add1/1
  ReductionCte/1 -> Product/2, Product1/2
  Product1/1 -> Add1/2
  Product/1 -> Add/2
  Add1/1 -> Tq_RL_out/1
  Add/1 -> Tq_RR_out/1
  Constant1/1 -> Flag_Power/1
  Constant/1 -> Flag_Temperature/1

== system TV_2021/If Action Subsystem1/VDC 2018 Complete/Constraints/Acelerating and braking without Regenerative/Control de Temperatura ==
  Tq_RR : Inport
  Tq_RL : Inport  Port=2
  ReductionCte : Inport  Port=3
  Action Port : ActionPort
  Add : Sum  Inputs=+-
  Add1 : Sum  Inputs=+-
  Constant : Constant
  Constant1 : Constant  Value=0
  Product : Product
  Product1 : Product
  Tq_RR_out : Outport
  Tq_RL_out : Outport  Port=2
  Flag_Temperature : Outport  Port=3
  Flag_Power : Outport  Port=4
  wires:
  Add/1 -> Tq_RR_out/1
  Add1/1 -> Tq_RL_out/1
  Product/1 -> Add/2
  Product1/1 -> Add1/2
  ReductionCte/1 -> Product1/2, Product/2
  Tq_RL/1 -> Add1/1, Product1/1
  Tq_RR/1 -> Add/1, Product/1
  Constant1/1 -> Flag_Power/1
  Constant/1 -> Flag_Temperature/1

== system TV_2021/If Action Subsystem1/VDC 2018 Complete/Constraints/Acelerating and braking without Regenerative/If Action 1 ==
  Trans_max_dynamic : Inport
  Action Port : ActionPort
  Trans_limit : Outport
  wires:
  Trans_max_dynamic/1 -> Trans_limit/1

== system TV_2021/If Action Subsystem1/VDC 2018 Complete/Constraints/Acelerating and braking without Regenerative/If Action 2 ==
  "Trans_max_static " : Inport
  Action Port : ActionPort
  Trans_limit : Outport
  wires:
  "Trans_max_static "/1 -> Trans_limit/1

== system TV_2021/If Action Subsystem1/VDC 2018 Complete/Constraints/Acelerating and braking without Regenerative/Momentum Z scaled ==
  Tq_RR_Lim : Inport
  Tq_RL_Lim : Inport  Port=2
  Tq_RR_wc : Inport  Port=3
  Tq_RL_wc : Inport  Port=4
  Tq_diff : Inport  Port=5
  MATLAB Function : MATLAB Function  TreatAsAtomicUnit=on
  Terminator3 : Terminator
  TQ_RR : Outport
  TQ_RL : Outport  Port=2
  wires:
  Tq_RL_Lim/1 -> MATLAB Function/2(tq_RL_lim)
  Tq_RR_Lim/1 -> MATLAB Function/1(tq_RR_lim)
  Tq_RR_wc/1 -> MATLAB Function/3(tq_RR_wc)
  Tq_RL_wc/1 -> MATLAB Function/4(tq_RL_wc)
  MATLAB Function/1(TQ_RR) -> TQ_RR/1
  MATLAB Function/2(TQ_RL) -> TQ_RL/1
  Tq_diff/1 -> Terminator3/1

== system TV_2021/If Action Subsystem1/VDC 2018 Complete/Constraints/Acelerating and braking without Regenerative/else ==
  Tq_RR : Inport
  Tq_RL : Inport  Port=2
  Action Port : ActionPort
  Constant : Constant  Value=0
  Constant1 : Constant  Value=0
  Tq_RR_out : Outport
  Tq_RL_out : Outport  Port=2
  Flag_Temperature : Outport  Port=3
  Flag_Power : Outport  Port=4
  wires:
  Tq_RR/1 -> Tq_RR_out/1
  Tq_RL/1 -> Tq_RL_out/1
  Constant1/1 -> Flag_Power/1
  Constant/1 -> Flag_Temperature/1

== system TV_2021/If Action Subsystem1/VDC 2018 Complete/Optimization SKF & CKF/Subsystem /CKF ==
  Derivative : Inport
  CKF_Initial : Inport  Port=2
  "CKF_prev " : Inport  Port=3
  Cte_CKF : Inport  Port=4
  Action Port : ActionPort
  If1 : If  IfExpression=u1 >= 900  ElseIfExpressions=u1 < 900  ShowElse=off
  Merge : Merge
  No spin : Subsystem  TreatAsAtomicUnit=on
  Saturation : Saturate  UpperLimit=1  LowerLimit=0.3
  "Spin " : Subsystem  TreatAsAtomicUnit=on
  "CKF_act " : Outport
  wires:
  Merge/1 -> Saturation/1
  "CKF_prev "/1 -> "Spin "/1(CKF_prev), No spin/2(CKF_prev)
  If1/1 -> "Spin "/Action
  Derivative/1 -> If1/1
  Cte_CKF/1 -> "Spin "/3(Cte_CKF)
  "Spin "/1("CKF_act1 ") -> Merge/2
  Saturation/1 -> "CKF_act "/1
  CKF_Initial/1 -> "Spin "/2("CKF_Initial "), No spin/1(CKF_Initial)
  If1/2 -> No spin/Action
  No spin/1(CKF_act0) -> Merge/1

== system TV_2021/If Action Subsystem1/VDC 2018 Complete/Optimization SKF & CKF/Subsystem /SKF ==
  Derivative : Inport
  "SKF_Initial " : Inport  Port=2
  SKF_prev : Inport  Port=3
  Cte_SKF : Inport  Port=4
  Action Port : ActionPort
  If : If  IfExpression=u1 >=900  ElseIfExpressions=u1 < 900  ShowElse=off
  Merge : Merge
  No spin : Subsystem  TreatAsAtomicUnit=on
  Saturation : Saturate  UpperLimit=1  LowerLimit=0.2
  Spin : Subsystem  TreatAsAtomicUnit=on
  SKF_act : Outport
  wires:
  Merge/1 -> Saturation/1
  Derivative/1 -> If/1
  Spin/1(SKF_act1) -> Merge/2
  "SKF_Initial "/1 -> Spin/1(SKF_Initial), No spin/1(SKF_Initial)
  No spin/1(SKF_act0) -> Merge/1
  If/2 -> No spin/Action
  SKF_prev/1 -> Spin/2(SKF_prev), No spin/2(SKF_prev)
  Cte_SKF/1 -> Spin/3(Cte_SKF)
  Saturation/1 -> SKF_act/1
  If/1 -> Spin/Action

== system TV_2021/If Action Subsystem1/VDC 2018 without Longitudinal/Constraints/Acelerating and braking without Regenerative/Control de Potencia  ==
  Tq_RR : Inport
  Tq_RL : Inport  Port=2
  ReductionCte : Inport  Port=3
  Action Port : ActionPort
  Add : Sum  Inputs=+-
  Add1 : Sum  Inputs=+-
  Product : Product
  Product1 : Product
  Tq_RR_out : Outport
  Tq_RL_out : Outport  Port=2
  wires:
  Tq_RR/1 -> Product/1, Add/1
  Tq_RL/1 -> Product1/1, Add1/1
  ReductionCte/1 -> Product/2, Product1/2
  Product1/1 -> Add1/2
  Product/1 -> Add/2
  Add1/1 -> Tq_RL_out/1
  Add/1 -> Tq_RR_out/1

== system TV_2021/If Action Subsystem1/VDC 2018 without Longitudinal/Constraints/Acelerating and braking without Regenerative/Control de Temperatura ==
  Tq_RR : Inport
  Tq_RL : Inport  Port=2
  ReductionCte : Inport  Port=3
  Action Port : ActionPort
  Add : Sum  Inputs=+-
  Add1 : Sum  Inputs=+-
  Product : Product
  Product1 : Product
  Tq_RR_out : Outport
  Tq_RL_out : Outport  Port=2
  wires:
  Add/1 -> Tq_RR_out/1
  Add1/1 -> Tq_RL_out/1
  Product/1 -> Add/2
  Product1/1 -> Add1/2
  ReductionCte/1 -> Product1/2, Product/2
  Tq_RL/1 -> Add1/1, Product1/1
  Tq_RR/1 -> Add/1, Product/1

== system TV_2021/If Action Subsystem1/VDC 2018 without Longitudinal/Constraints/Acelerating and braking without Regenerative/If Action 1 ==
  Trans_max_dynamic : Inport
  Action Port : ActionPort
  Trans_limit : Outport
  wires:
  Trans_max_dynamic/1 -> Trans_limit/1

== system TV_2021/If Action Subsystem1/VDC 2018 without Longitudinal/Constraints/Acelerating and braking without Regenerative/If Action 2 ==
  "Trans_max_static " : Inport
  Action Port : ActionPort
  Trans_limit : Outport
  wires:
  "Trans_max_static "/1 -> Trans_limit/1

== system TV_2021/If Action Subsystem1/VDC 2018 without Longitudinal/Constraints/Acelerating and braking without Regenerative/Momentum Z scaled ==
  Tq_RR_Lim : Inport
  Tq_RL_Lim : Inport  Port=2
  Tq_RR_wc : Inport  Port=3
  Tq_RL_wc : Inport  Port=4
  MATLAB Function : MATLAB Function  TreatAsAtomicUnit=on
  TQ_RR : Outport
  TQ_RL : Outport  Port=2
  wires:
  Tq_RL_Lim/1 -> MATLAB Function/2(tq_RL_lim)
  Tq_RR_Lim/1 -> MATLAB Function/1(tq_RR_lim)
  Tq_RR_wc/1 -> MATLAB Function/3(tq_RR_wc)
  Tq_RL_wc/1 -> MATLAB Function/4(tq_RL_wc)
  MATLAB Function/1(TQ_RR) -> TQ_RR/1
  MATLAB Function/2(TQ_RL) -> TQ_RL/1

== system TV_2021/If Action Subsystem1/VDC 2018 without Longitudinal/Constraints/Acelerating and braking without Regenerative/else ==
  Tq_RR : Inport
  Tq_RL : Inport  Port=2
  Action Port : ActionPort
  Tq_RR_out : Outport
  Tq_RL_out : Outport  Port=2
  wires:
  Tq_RR/1 -> Tq_RR_out/1
  Tq_RL/1 -> Tq_RL_out/1

== system TV_2021/If Action Subsystem1/VDC 2018 without Longitudinal/Optimization SKF & CKF/Subsystem /CKF ==
  Derivative : Inport
  CKF_Initial : Inport  Port=2
  "CKF_prev " : Inport  Port=3
  Cte_CKF : Inport  Port=4
  If1 : If  IfExpression=u1 >= 900  ElseIfExpressions=u1 < 900  ShowElse=off
  Merge : Merge
  No spin : Subsystem  TreatAsAtomicUnit=on
  Saturation : Saturate  UpperLimit=1  LowerLimit=0.3
  "Spin " : Subsystem  TreatAsAtomicUnit=on
  "CKF_act " : Outport
  wires:
  Merge/1 -> Saturation/1
  "CKF_prev "/1 -> "Spin "/1(CKF_prev), No spin/2(CKF_prev)
  Derivative/1 -> If1/1
  Cte_CKF/1 -> "Spin "/3(Cte_CKF)
  "Spin "/1("CKF_act1 ") -> Merge/2
  Saturation/1 -> "CKF_act "/1
  CKF_Initial/1 -> "Spin "/2("CKF_Initial "), No spin/1(CKF_Initial)
  If1/2 -> No spin/Action
  No spin/1(CKF_act0) -> Merge/1
  If1/1 -> "Spin "/Action

== system TV_2021/Vehicle Dynamics Control 1/Steering TV 2017 with TC/Constraints/current_limitation1/constants_saturator ==
  note: Saturamos con unos
      | valores máximos
      | preestablecidos
  allowed_current [%] : Inport
  max_discharge_current : Inport  Port=2
  max_regen_current : Inport  Port=3
  Constant : Constant  Value=0
  Gain2 : Gain  Gain=-1
  Saturation Dynamic : simulink/Discontinuities/Saturation Dynamic  OutMin=[]  OutMax=[]  OutDataTypeStr=Inherit: Same as second input  OutDataType=fixdt(1, 16)  OutScaling=2^-10  DoSatur=off
  Saturation Dynamic1 : simulink/Discontinuities/Saturation Dynamic  OutMin=[]  OutMax=[]  OutDataTypeStr=Inherit: Same as second input  OutDataType=fixdt(1, 16)  OutScaling=2^-10  DoSatur=off
  limited_discharge_actual : Outport  VectorParamsAs1DForOutWhenUnconnected=on
  limited_regen_actual : Outport  Port=2  VectorParamsAs1DForOutWhenUnconnected=on
  wires:
  max_discharge_current/1 -> Saturation Dynamic/1
  Saturation Dynamic/1 -> limited_discharge_actual/1
  allowed_current [%]/1 -> Gain2/1, Saturation Dynamic/2
  Saturation Dynamic1/1 -> limited_regen_actual/1
  Gain2/1 -> Saturation Dynamic1/2
  Constant/1 -> Saturation Dynamic1/3, Saturation Dynamic/3
  max_regen_current/1 -> Saturation Dynamic1/1

== system TV_2021/Vehicle Dynamics Control 1/Steering TV 2017 with TC/Constraints/current_limitation1/temperature_rise_limitator ==
  note: output 0 si está por
      | debajo de 50ºC, 1 si está
      | por encima
  note: Se limita la corriente en proporción
      | al ratio entre la temperatura actual y 50ºC
  note: magia chunga para
      | que los números cuadren
  note: saturamos de 1 a 0 por si acaso
  note: initial_limitation es una constante para la reducción inicial (de 0 a 1, más bajo significa que cambia
      | menos, más alto la limitación
      | inicial es más bestia).
  max_cell_temp : Inport
  initial_limitation : Inport  Port=2
  Add1 : Sum  Inputs=-+
  Add2 : Sum  Inputs=-++
  Add3 : Sum  Inputs=+-
  Constant1 : Constant  Value=55
  Constant2 : Constant  Value=5
  Constant3 : Constant
  Divide : Product  Inputs=*/
  Product4 : Product
  Saturation1 : Saturate  UpperLimit=1  LowerLimit=0
  Scope2 : Scope
  Scope4 : Scope
  Temp higher than 50 : simulink/Logic and Bit Operations/Compare To Constant  relop=>=  const=50  OutDataTypeStr=boolean  ZeroCross=off
  allowed_current : Outport  VectorParamsAs1DForOutWhenUnconnected=on
  wires:
  initial_limitation/1 -> Add3/2
  Saturation1/1 -> allowed_current/1
  Add1/1 -> Divide/2
  Add3/1 -> Product4/1
  Add2/1 -> Saturation1/1, Scope2/1
  Product4/1 -> Add2/2
  Constant2/1 -> Add1/1
  Temp higher than 50/1 -> Product4/2, Add2/1
  max_cell_temp/1 -> Temp higher than 50/1, Scope4/1, Add1/2
  Constant1/1 -> Divide/1
  Constant3/1 -> Add2/3
  Divide/1 -> Add3/1

== system TV_2021/Vehicle Dynamics Control 1/Steering TV 2017 with TC/Optimization SKF & CKF/Subsystem /CKF ==
  Derivative : Inport
  CKF_Initial : Inport  Port=2
  "CKF_prev " : Inport  Port=3
  Cte_CKF : Inport  Port=4
  Action Port : ActionPort
  If1 : If  IfExpression=u1 >= 900  ElseIfExpressions=u1 < 900  ShowElse=off
  Merge : Merge
  No spin : Subsystem  TreatAsAtomicUnit=on
  Saturation : Saturate  UpperLimit=1  LowerLimit=0.3
  "Spin " : Subsystem  TreatAsAtomicUnit=on
  "CKF_act " : Outport
  wires:
  Derivative/1 -> If1/1
  No spin/1(CKF_act0) -> Merge/1
  If1/2 -> No spin/Action
  CKF_Initial/1 -> No spin/1(CKF_Initial), "Spin "/2("CKF_Initial ")
  Saturation/1 -> "CKF_act "/1
  "Spin "/1("CKF_act1 ") -> Merge/2
  Cte_CKF/1 -> "Spin "/3(Cte_CKF)
  If1/1 -> "Spin "/Action
  "CKF_prev "/1 -> No spin/2(CKF_prev), "Spin "/1(CKF_prev)
  Merge/1 -> Saturation/1

== system TV_2021/Vehicle Dynamics Control 1/Steering TV 2017 with TC/Optimization SKF & CKF/Subsystem /SKF ==
  Derivative : Inport
  "SKF_Initial " : Inport  Port=2
  SKF_prev : Inport  Port=3
  Cte_SKF : Inport  Port=4
  Action Port : ActionPort
  Display : Display
  Display1 : Display
  If : If  IfExpression=u1 >=900  ElseIfExpressions=u1 < 900  ShowElse=off
  Merge : Merge
  No spin : Subsystem  TreatAsAtomicUnit=on
  Saturation : Saturate  UpperLimit=1  LowerLimit=0.3
  Spin : Subsystem  TreatAsAtomicUnit=on
  SKF_act : Outport
  wires:
  Derivative/1 -> If/1
  If/1 -> Spin/Action
  Saturation/1 -> SKF_act/1, Display1/1
  Cte_SKF/1 -> Spin/3(Cte_SKF)
  SKF_prev/1 -> No spin/2(SKF_prev), Spin/2(SKF_prev), Display/1
  If/2 -> No spin/Action
  No spin/1(SKF_act0) -> Merge/1
  "SKF_Initial "/1 -> No spin/1(SKF_Initial), Spin/1(SKF_Initial)
  Spin/1(SKF_act1) -> Merge/2
  Merge/1 -> Saturation/1

== system TV_2021/Vehicle Dynamics Control 1/VDC 2018 Complete/Constraints/Acelerating and braking without Regenerative/Control de Potencia  ==
  Tq_RR : Inport
  Tq_RL : Inport  Port=2
  ReductionCte : Inport  Port=3
  Action Port : ActionPort
  Add : Sum  Inputs=+-
  Add1 : Sum  Inputs=+-
  Constant : Constant  Value=0
  Constant1 : Constant
  Product : Product
  Product1 : Product
  Tq_RR_out : Outport
  Tq_RL_out : Outport  Port=2
  Flag_Temperature : Outport  Port=3
  Flag_Power : Outport  Port=4
  wires:
  Constant/1 -> Flag_Temperature/1
  Constant1/1 -> Flag_Power/1
  Add/1 -> Tq_RR_out/1
  Add1/1 -> Tq_RL_out/1
  Product/1 -> Add/2
  Product1/1 -> Add1/2
  ReductionCte/1 -> Product1/2, Product/2
  Tq_RL/1 -> Add1/1, Product1/1
  Tq_RR/1 -> Add/1, Product/1

== system TV_2021/Vehicle Dynamics Control 1/VDC 2018 Complete/Constraints/Acelerating and braking without Regenerative/Control de Temperatura ==
  Tq_RR : Inport
  Tq_RL : Inport  Port=2
  ReductionCte : Inport  Port=3
  Action Port : ActionPort
  Add : Sum  Inputs=+-
  Add1 : Sum  Inputs=+-
  Constant : Constant
  Constant1 : Constant  Value=0
  Product : Product
  Product1 : Product
  Tq_RR_out : Outport
  Tq_RL_out : Outport  Port=2
  Flag_Temperature : Outport  Port=3
  Flag_Power : Outport  Port=4
  wires:
  Constant/1 -> Flag_Temperature/1
  Constant1/1 -> Flag_Power/1
  Tq_RR/1 -> Product/1, Add/1
  Tq_RL/1 -> Product1/1, Add1/1
  ReductionCte/1 -> Product/2, Product1/2
  Product1/1 -> Add1/2
  Product/1 -> Add/2
  Add1/1 -> Tq_RL_out/1
  Add/1 -> Tq_RR_out/1

== system TV_2021/Vehicle Dynamics Control 1/VDC 2018 Complete/Constraints/Acelerating and braking without Regenerative/If Action 1 ==
  Trans_max_dynamic : Inport
  Action Port : ActionPort
  Trans_limit : Outport
  wires:
  Trans_max_dynamic/1 -> Trans_limit/1

== system TV_2021/Vehicle Dynamics Control 1/VDC 2018 Complete/Constraints/Acelerating and braking without Regenerative/If Action 2 ==
  "Trans_max_static " : Inport
  Action Port : ActionPort
  Trans_limit : Outport
  wires:
  "Trans_max_static "/1 -> Trans_limit/1

== system TV_2021/Vehicle Dynamics Control 1/VDC 2018 Complete/Constraints/Acelerating and braking without Regenerative/Momentum Z scaled ==
  Tq_RR_Lim : Inport
  Tq_RL_Lim : Inport  Port=2
  Tq_RR_wc : Inport  Port=3
  Tq_RL_wc : Inport  Port=4
  Tq_diff : Inport  Port=5
  Display : Display
  Display1 : Display
  MATLAB Function : MATLAB Function  TreatAsAtomicUnit=on
  TQ_RR : Outport
  TQ_RL : Outport  Port=2
  wires:
  Tq_diff/1 -> MATLAB Function/5(tq_diff)
  MATLAB Function/2(TQ_RL) -> TQ_RL/1, Display1/1
  MATLAB Function/1(TQ_RR) -> TQ_RR/1, Display/1
  Tq_RL_wc/1 -> MATLAB Function/4(tq_RL_wc)
  Tq_RR_wc/1 -> MATLAB Function/3(tq_RR_wc)
  Tq_RR_Lim/1 -> MATLAB Function/1(tq_RR_lim)
  Tq_RL_Lim/1 -> MATLAB Function/2(tq_RL_lim)

== system TV_2021/Vehicle Dynamics Control 1/VDC 2018 Complete/Constraints/Acelerating and braking without Regenerative/else ==
  Tq_RR : Inport
  Tq_RL : Inport  Port=2
  Action Port : ActionPort
  Constant : Constant  Value=0
  Constant1 : Constant  Value=0
  Tq_RR_out : Outport
  Tq_RL_out : Outport  Port=2
  Flag_Temperature : Outport  Port=3
  Flag_Power : Outport  Port=4
  wires:
  Constant/1 -> Flag_Temperature/1
  Constant1/1 -> Flag_Power/1
  Tq_RL/1 -> Tq_RL_out/1
  Tq_RR/1 -> Tq_RR_out/1

== system TV_2021/Vehicle Dynamics Control 1/VDC 2018 Complete/Lateral Dynamics/Tire Longitudinal Force Difference/ Momentum_Z to Longitudinal Force Difference ==
  "\tMomentumZ [Nm]" : Inport
  RearTrackwidth [m] : Inport  Port=2
  Constant : Constant  Value=2
  Divide : Product  Inputs=*/
  Divide1 : Product  Inputs=*/
  Fx_diff [N] : Outport
  wires:
  RearTrackwidth [m]/1 -> Divide1/1
  Constant/1 -> Divide1/2
  "\tMomentumZ [Nm]"/1 -> Divide/1
  Divide1/1 -> Divide/2
  Divide/1 -> Fx_diff [N]/1

== system TV_2021/Vehicle Dynamics Control 1/VDC 2018 Complete/Lateral Dynamics/Tire Longitudinal Force Difference/Momentum respect to Z-axis to correct the error ==
  Yaw_error_[º/s] : Inport
  Iz [kg/m^3] : Inport  Port=2
  Correction_Time [s] : Inport  Port=3
  Divide : Product  Inputs=*/
  Product : Product
  Momentum_Z [Nm] : Outport
  wires:
  Iz [kg/m^3]/1 -> Product/2
  Yaw_error_[º/s]/1 -> Product/1
  Product/1 -> Divide/1
  Correction_Time [s]/1 -> Divide/2
  Divide/1 -> Momentum_Z [Nm]/1

== system TV_2021/Vehicle Dynamics Control 1/VDC 2018 Complete/Optimization SKF & CKF/Subsystem /CKF ==
  Derivative : Inport
  CKF_Initial : Inport  Port=2
  "CKF_prev " : Inport  Port=3
  Cte_CKF : Inport  Port=4
  Action Port : ActionPort
  If1 : If  IfExpression=u1 >= 900  ElseIfExpressions=u1 < 900  ShowElse=off
  Merge : Merge
  No spin : Subsystem  TreatAsAtomicUnit=on
  Saturation : Saturate  UpperLimit=1  LowerLimit=0.3
  "Spin " : Subsystem  TreatAsAtomicUnit=on
  "CKF_act " : Outport
  wires:
  No spin/1(CKF_act0) -> Merge/1
  If1/2 -> No spin/Action
  CKF_Initial/1 -> No spin/1(CKF_Initial), "Spin "/2("CKF_Initial ")
  Saturation/1 -> "CKF_act "/1
  "Spin "/1("CKF_act1 ") -> Merge/2
  Cte_CKF/1 -> "Spin "/3(Cte_CKF)
  Derivative/1 -> If1/1
  If1/1 -> "Spin "/Action
  "CKF_prev "/1 -> No spin/2(CKF_prev), "Spin "/1(CKF_prev)
  Merge/1 -> Saturation/1

== system TV_2021/Vehicle Dynamics Control 1/VDC 2018 Complete/Optimization SKF & CKF/Subsystem /SKF ==
  Derivative : Inport
  "SKF_Initial " : Inport  Port=2
  SKF_prev : Inport  Port=3
  Cte_SKF : Inport  Port=4
  Action Port : ActionPort
  Display : Display
  If : If  IfExpression=u1 >=900  ElseIfExpressions=u1 < 900  ShowElse=off
  Merge : Merge
  No spin : Subsystem  TreatAsAtomicUnit=on
  Saturation : Saturate  UpperLimit=1  LowerLimit=0.3
  Spin : Subsystem  TreatAsAtomicUnit=on
  SKF_act : Outport
  wires:
  If/1 -> Spin/Action
  Saturation/1 -> SKF_act/1
  Cte_SKF/1 -> Spin/3(Cte_SKF)
  SKF_prev/1 -> No spin/2(SKF_prev), Spin/2(SKF_prev)
  If/2 -> No spin/Action
  No spin/1(SKF_act0) -> Merge/1
  "SKF_Initial "/1 -> No spin/1(SKF_Initial), Spin/1(SKF_Initial)
  Spin/1(SKF_act1) -> Merge/2
  Derivative/1 -> Display/1, If/1
  Merge/1 -> Saturation/1

== system TV_2021/Vehicle Dynamics Control 1/VDC 2018 without Longitudinal/Constraints/Acelerating and braking without Regenerative/Control de Potencia 1 ==
  Tq_RR : Inport
  Tq_RL : Inport  Port=2
  ReductionCte : Inport  Port=3
  Action Port : ActionPort
  Add : Sum  Inputs=+-
  Add1 : Sum  Inputs=+-
  Product : Product
  Product1 : Product
  Tq_RR_out : Outport
  Tq_RL_out : Outport  Port=2
  wires:
  Add/1 -> Tq_RR_out/1
  Add1/1 -> Tq_RL_out/1
  Product/1 -> Add/2
  Product1/1 -> Add1/2
  ReductionCte/1 -> Product1/2, Product/2
  Tq_RL/1 -> Add1/1, Product1/1
  Tq_RR/1 -> Add/1, Product/1

== system TV_2021/Vehicle Dynamics Control 1/VDC 2018 without Longitudinal/Constraints/Acelerating and braking without Regenerative/Control de Temperatura1 ==
  Tq_RR : Inport
  Tq_RL : Inport  Port=2
  ReductionCte : Inport  Port=3
  Action Port : ActionPort
  Add : Sum  Inputs=+-
  Add1 : Sum  Inputs=+-
  Product : Product
  Product1 : Product
  Tq_RR_out : Outport
  Tq_RL_out : Outport  Port=2
  wires:
  Add/1 -> Tq_RR_out/1
  ReductionCte/1 -> Product/2, Product1/2
  Tq_RL/1 -> Product1/1, Add1/1
  Tq_RR/1 -> Product/1, Add/1
  Add1/1 -> Tq_RL_out/1
  Product1/1 -> Add1/2
  Product/1 -> Add/2

== system TV_2021/Vehicle Dynamics Control 1/VDC 2018 without Longitudinal/Constraints/Acelerating and braking without Regenerative/If Action 1 ==
  Trans_max_dynamic : Inport
  Action Port : ActionPort
  Trans_limit : Outport
  wires:
  Trans_max_dynamic/1 -> Trans_limit/1

== system TV_2021/Vehicle Dynamics Control 1/VDC 2018 without Longitudinal/Constraints/Acelerating and braking without Regenerative/If Action 2 ==
  "Trans_max_static " : Inport
  Action Port : ActionPort
  Trans_limit : Outport
  wires:
  "Trans_max_static "/1 -> Trans_limit/1

== system TV_2021/Vehicle Dynamics Control 1/VDC 2018 without Longitudinal/Constraints/Acelerating and braking without Regenerative/Momentum Z scaled ==
  Tq_RR_Lim : Inport
  Tq_RL_Lim : Inport  Port=2
  Tq_RR_wc : Inport  Port=3
  Tq_RL_wc : Inport  Port=4
  MATLAB Function : MATLAB Function  TreatAsAtomicUnit=on
  TQ_RR : Outport
  TQ_RL : Outport  Port=2
  wires:
  MATLAB Function/2(TQ_RL) -> TQ_RL/1
  MATLAB Function/1(TQ_RR) -> TQ_RR/1
  Tq_RL_wc/1 -> MATLAB Function/4(tq_RL_wc)
  Tq_RR_wc/1 -> MATLAB Function/3(tq_RR_wc)
  Tq_RR_Lim/1 -> MATLAB Function/1(tq_RR_lim)
  Tq_RL_Lim/1 -> MATLAB Function/2(tq_RL_lim)

== system TV_2021/Vehicle Dynamics Control 1/VDC 2018 without Longitudinal/Constraints/Acelerating and braking without Regenerative/else1 ==
  Tq_RR : Inport
  Tq_RL : Inport  Port=2
  Action Port : ActionPort
  Tq_RR_out : Outport
  Tq_RL_out : Outport  Port=2
  wires:
  Tq_RL/1 -> Tq_RL_out/1
  Tq_RR/1 -> Tq_RR_out/1

== system TV_2021/Vehicle Dynamics Control 1/VDC 2018 without Longitudinal/Optimization SKF & CKF/Subsystem /CKF ==
  Derivative : Inport
  CKF_Initial : Inport  Port=2
  "CKF_prev " : Inport  Port=3
  Cte_CKF : Inport  Port=4
  If1 : If  IfExpression=u1 >= 900  ElseIfExpressions=u1 < 900  ShowElse=off
  Merge : Merge
  No spin : Subsystem  TreatAsAtomicUnit=on
  Saturation : Saturate  UpperLimit=1  LowerLimit=0.3
  "Spin " : Subsystem  TreatAsAtomicUnit=on
  "CKF_act " : Outport
  wires:
  If1/1 -> "Spin "/Action
  No spin/1(CKF_act0) -> Merge/1
  If1/2 -> No spin/Action
  CKF_Initial/1 -> No spin/1(CKF_Initial), "Spin "/2("CKF_Initial ")
  Saturation/1 -> "CKF_act "/1
  "Spin "/1("CKF_act1 ") -> Merge/2
  Cte_CKF/1 -> "Spin "/3(Cte_CKF)
  Derivative/1 -> If1/1
  "CKF_prev "/1 -> No spin/2(CKF_prev), "Spin "/1(CKF_prev)
  Merge/1 -> Saturation/1
